simulink model "PQ_2V"  (R2023a)
settings: Solver=FixedStepAuto  StartTime=0.0  StopTime=10.0  FixedStep=Ts  RelTol=1e-3
InitFcn:
  | Ts = 1e-6;
  | Ikp = 0.1 ;
  | Iki = 0.002*12800 ;
  | 
  | Pref = 0;
  | Qref = 600e3;
libraries: slpidlib x4, spsabctodq0Lib x3, spsThreePhaseSeriesRLCBranchLib x2, spsThreePhaseVIMeasurementLib x1, spsDCVoltageSourceLib x1, powerlib_extras x1, spsGroundLib x1, spsMultimeterLib x1, spsPLL3phLib x1, spsPower3phInstantaneousLib x1, spsSeriesRLCBranchLib x1, spsThreePhaseSourceLib x1
settings Model: Creator=Cyril  LastModifiedBy=Cyril
settings SolverCC: AlgebraicLoopSolver=TrustRegion
settings DebuggingCC: UnconnectedInputMsg=warning  UnconnectedOutputMsg=warning  UnconnectedLineMsg=warning
settings ModelReferenceCC: EnableRefExpFcnMdlSchedulingChecks=on
settings RTWCC: DLArmComputeVersion=19.05

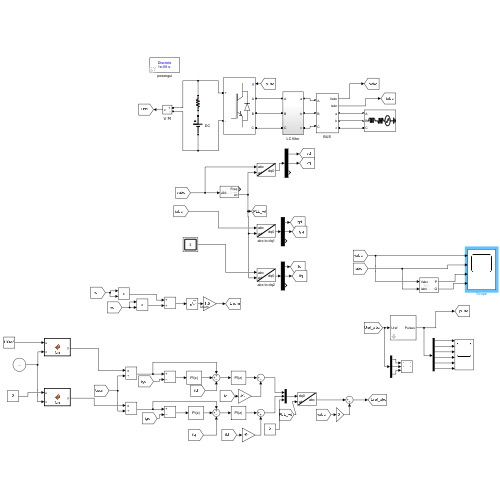
[thumbnail: Simulink's stored preview of the top-level diagram]
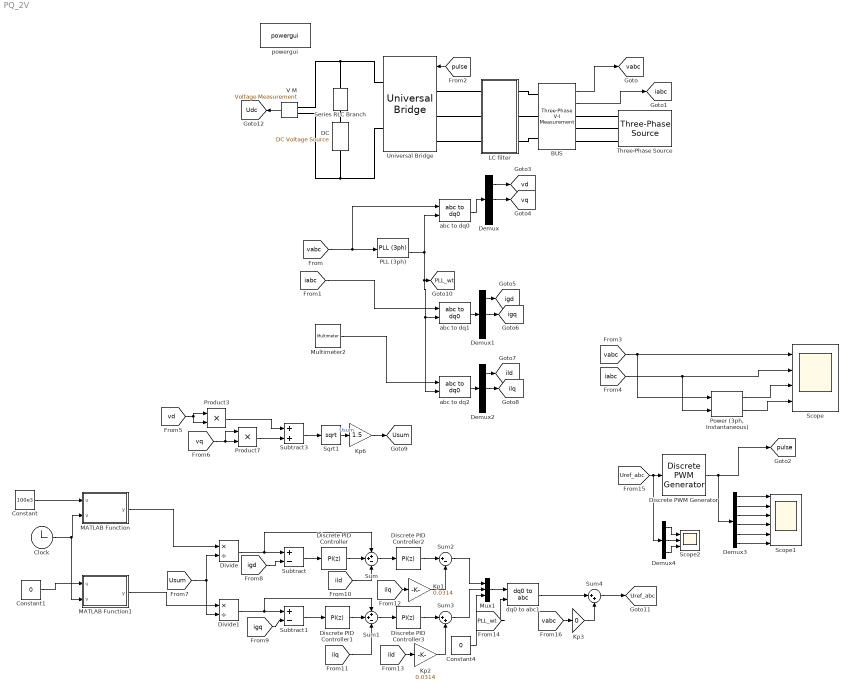
== system PQ_2V ==
  BUS : spsThreePhaseVIMeasurementLib/Three-Phase V-I Measurement  VoltageMeasurement=phase-to-ground  SetLabelV=off  LabelV=Vabc  Vpu=off  VpuLL=off  CurrentMeasurement=yes  SetLabelI=off  LabelI=Iabc  Ipu=off  Pbase=100e6  Vbase=500e3  OutputType=Complex  PhasorSimulation=off  PSBequivalent=0
  Clock : Clock
  Constant : Constant  Value=100e3  SampleTime=-1
  Constant1 : Constant  Value=0  SampleTime=-1
  Constant4 : Constant  Value=0
  "DC " : spsDCVoltageSourceLib/DC Voltage Source  Amplitude=800  Measurements=None
  Demux{,1..2,4} (4 alike) : Demux  Outputs=3
  Demux3 : Demux  Outputs=6
  Discrete PWM Generator : powerlib_extras/Discrete  Control Blocks/Discrete PWM Generator  GeneratorMode="3-arm  bridge (6 pulses)"  Fc=4266  Ts=Ts  Internal=off  mIndex=0.4  Freq=60  Phase=0
  Discrete PID Controller{,1..3} (4 alike) : slpidlib/PID Controller  Controller=PI  Form=Parallel  TimeDomain=Discrete-time  UseExternalTs=off  SampleTime=Ts  IntegratorMethod=Forward Euler  FilterMethod=Forward Euler  ControllerParametersSource=internal  P=Ikp  I=Iki  UseKiTs=off  D=0  N=100  UseFilter=on  TunerSelectOption=Transfer Function Based (PID Tuner App)  InitialConditionSource=internal  InitialConditionForIntegrator=0  InitialConditionForFilter=0  DifferentiatorICPrevScaledInput=0  ExternalReset=none  TrackingMode=off  Kt=1  LimitOutput=off  SatLimitsSource=internal  UpperSaturationLimit=inf  LowerSaturationLimit=-inf  LinearizeAsGain=off  AntiWindupMode=none  Kb=1  LimitIntegrator=off  UpperIntegratorSaturationLimit=inf  LowerIntegratorSaturationLimit=-inf  POutMin=[]  POutMax=[]  IOutMin=[]  IOutMax=[]  DOutMin=[]  DOutMax=[]  NOutMin=[]  NOutMax=[]  SumOutMin=[]  SumOutMax=[]  SaturationOutMin=[]  SaturationOutMax=[]  PParamMin=[]  PParamMax=[]  IParamMin=[]  IParamMax=[]  DParamMin=[]  DParamMax=[]  NParamMin=[]  NParamMax=[]  KbParamMin=[]  KbParamMax=[]  KtParamMin=[]  KtParamMax=[]  KbOutMin=[]  KbOutMax=[]  KtOutMin=[]  KtOutMax=[]  IntegratorOutMin=[]  IntegratorOutMax=[]  FilterOutMin=[]  FilterOutMax=[]  SumI1OutMin=[]  SumI1OutMax=[]  SumI2OutMin=[]  SumI2OutMax=[]  SumI3OutMin=[]  SumI3OutMax=[]  SumI4OutMin=[]  SumI4OutMax=[]  SumDOutMin=[]  SumDOutMax=[]  DifferentiatorOutMin=[]  DifferentiatorOutMax=[]  FilterDiffOutCoefMin=[]  FilterDiffOutCoefMax=[]  ReciprocalOutMin=[]  ReciprocalOutMax=[]  SumDenOutMin=[]  SumDenOutMax=[]  SumNumOutMin=[]  SumNumOutMax=[]  DivideOutMin=[]  DivideOutMax=[]  UdiffTsProdOutMin=[]  UdiffTsProdOutMax=[]  NTsProdOutMin=[]  NTsProdOutMax=[]  UintegralTsProdOutMin=[]  UintegralTsProdOutMax=[]  UngainTsProdOutMin=[]  UngainTsProdOutMax=[]  ClampingZeroOutDataTypeStr=Inherit: Inherit via back propagation  ClampingZeroOutMin=[]  ClampingZeroOutMax=[]  FilterDenConstantOutDataTypeStr=Inherit: Inherit via back propagation  FilterDenConstantOutMin=[]  FilterDenConstantOutMax=[]  PCopyOutDataTypeStr=Inherit: Inherit via back propagation  PCopyOutMin=[]  PCopyOutMax=[]  NCopyOutDataTypeStr=Inherit: Inherit via back propagation  NCopyOutMin=[]  NCopyOutMax=[]  IntegratorContinuousStateAttributes=''  IntegratorStateMustResolveToSignalObject=off  IntegratorRTWStateStorageClass=Auto  FilterContinuousStateAttributes=''  FilterStateMustResolveToSignalObject=off  FilterRTWStateStorageClass=Auto  ParallelPVariant=InternalParameters  IdealPVariant=Disabled  IVariant=InternalParameters  DVariant=Disabled  IntegratorVariant=Discrete  SatVariant=Disabled  AWVariant=Passthrough  PCopyVariant=Disabled  TRVariant=Disabled  FdbkBlocksVariant=Forward  IdealPFdbkVariant=Disabled  SatFdbkVariant=Disabled  DerivativeFilterVariant=Disabled  NVariant=Disabled  NCopyVariant=Disabled_SignalSpec  FilterICVariant=Disabled  IntegratorICVariant=InternalICs  ExternalResetVariant=Disabled  TRSumVariant=Passthrough  SumFdbkVariant=Disabled  SumVariant=Sum_PI  TsampFilterVariant=InternalTs  TsampNgainVariant=Passthrough  TsampIntegralVariant=Disabled_SignalSpec  ExternalSaturationOutDataTypeStr=Inherit: Same as second input
  Divide : Product  Inputs=*/
  Divide1 : Product  Inputs=*/
  Kp1 : Gain  Gain=0.0314  SaturateOnIntegerOverflow=on  OutDataTypeStr=Inherit: Same as input  ParamDataTypeStr=Inherit: Same as input
  Kp2 : Gain  Gain=0.0314  SaturateOnIntegerOverflow=on  OutDataTypeStr=Inherit: Same as input  ParamDataTypeStr=Inherit: Same as input
  Kp3 : Gain  Gain=0  SaturateOnIntegerOverflow=on  OutDataTypeStr=Inherit: Same as input  ParamDataTypeStr=Inherit: Same as input
  Kp6 : Gain  Gain=1.5  SaturateOnIntegerOverflow=on  OutDataTypeStr=Inherit: Same as input  ParamDataTypeStr=Inherit: Same as input
  LC filter : Subsystem
  MATLAB Function : MATLAB Function  TreatAsAtomicUnit=on
  MATLAB Function1 : MATLAB Function  TreatAsAtomicUnit=on
  Multimeter2 : spsMultimeterLib/Multimeter  L=3  sel=[1 2 3]  Gain=[1 1 1]  OutputType=Complex  PlotAtSimulationStop=off  PhasorSimulation=off
  Mux1 : Mux  Inputs=3
  PLL (3ph) : spsPLL3phLib/PLL (3ph)  Fmin=50  Par_Init=[0, 50]  ParK=[180, 3200, 1]  TcD=1e-5  MaxRateChangeFreq=12  FilterCutOffFreq=25  Ts=Ts  AGC=on
  "Power (3ph, Instantaneous)" : spsPower3phInstantaneousLib/Power (3ph, Instantaneous)
  Product3 : Product
  Product7 : Product
  Scope : Scope  NumInputPorts=4
  Scope1 : Scope  NumInputPorts=6
  Scope2 : Scope  NumInputPorts=3
  Series RLC Branch : spsSeriesRLCBranchLib/Series RLC Branch  LConnTagsString=__new0  RConnTagsString=__new0  BranchType=R  Resistance=1e-4  Inductance=1e-3  SetiL0=off  InitialCurrent=0  Capacitance=1e-6  Setx0=off  InitialVoltage=0  Measurements=None
  Sqrt1 : Sqrt
  Subtract : Sum  Inputs=+-
  Subtract1 : Sum  Inputs=+-
  Subtract3 : Sum
  Sum : Sum  Inputs=++-
  Sum1 : Sum  Inputs=++-
  Sum2 : Sum  Inputs=|+-
  Sum3 : Sum  Inputs=|++
  Sum4 : Sum  Inputs=|++
  Three-Phase Source : spsThreePhaseSourceLib/Three-Phase Source  InternalConnection=Yg  VoltagePhases=off  Voltage=380  PhaseAngle=0  Voltage_phases=[25e3 25e3 25e3]/sqrt(3)  PhaseAngles_phases=[0 -120 +120]  Frequency=50  NonIdealSource=on  SpecifyImpedance=on  Resistance=0.8929  Inductance=16.58e-3  ShortCircuitLevel=5000e6  BaseVoltage=380  XRratio=7  BusType=swing  Pref=0  Qref=0  Prefabc=[10e3, 10e3, 10e3]  Qrefabc=[0, 0, 0]  Qmin=-inf  Qmax=inf
  Universal Bridge : spsUniversalBridgeLib/Universal Bridge  Arms=3  SnubberResistance=1e5  SnubberCapacitance=inf  Device=IGBT / Diodes  Ron=1e-3  Lon=0  ForwardVoltages="[1  1]"  ForwardVoltage=0  GTOparameters=[ 10e-6 , 20e-6 ]  IGBTparameters=[ 1e-6 , 2e-6 ]  Measurements=None  Measurements_2=None  converterType=Rectifier
  V M : spsVoltageMeasurementLib/Voltage Measurement  PhasorSimulation=off  OutputType=Complex  PSBequivalent=0
  abc to dq0 : spsabctodq0Lib/abc to dq0  Alignment=90 degrees behind phase A axis
  abc to dq1 : spsabctodq0Lib/abc to dq0  Alignment=90 degrees behind phase A axis
  abc to dq2 : spsabctodq0Lib/abc to dq0  Alignment=90 degrees behind phase A axis
  dq0 to abc1 : spsdq0toabcLib/dq0 to abc  Alignment=90 degrees behind phase A axis
  powergui : sps_lib/powergui  Priority=1  SimulationMode=Discrete  SampleTime=Ts  frequency=60  Iterations=50  frequencyindice=50  Pbase=100e6  ErrMax=1e-4  UnitsV=kV  UnitsW=MW  buscounter=0  FunctionMessages=off  echomessages=off  EnableUseOfTLC=off  CurrentSourceSwitches=off  DisableSnubberDevices=off  DisableRonSwitches=off  DisableVfSwitches=off  DisplayEquations=off  AutomaticDiscreteSolvers=off  SolverType=Tustin/Backward Euler (TBE)  Interpol=off  ExternalGateDelay=off  methode=off  Ts=100  x0status=blocks  SPID=on  SwTol=0  HookPort=off  NonlinearTolerance=1e-4  nMaxIteration=100  ContinueOnMaxIteration=off  RestoreLinks=warning  ResistiveCurrentMeasurement=off  Frange=[0:2:500]  Ylog=off  Xlog=on  ShowGrid=off  save=off  variable=ZData  structure=0  ZoomFFT=off  StartTime=0.0  cycles=1  DisplayStyle=1  fundamental=60  FreqAxis=off  MaxFrequency=1000  frequencyindicesteady=1  RmsSteady=1  display=off
  tag scope: PLL_wt=global, Udc=global, Uref_abc=global, Usum=global, iabc=global, igd=global, igq=global, ild=global, ilq=global, pulse=global, vabc=global, vd=global, vq=global
  wires:
  BUS/1 -> [vabc]
  BUS/2 -> [iabc]
  [vabc] -> abc to dq0/1, PLL (3ph)/1
  PLL (3ph)/2 -> [PLL_wt], abc to dq2/2, abc to dq1/2, abc to dq0/2
  [iabc] -> abc to dq1/1
  Discrete PWM Generator/1 -> Demux3/1, [pulse]
  [pulse] -> Universal Bridge/1
  [vabc] -> "Power (3ph, Instantaneous)"/1, Scope/1
  [iabc] -> "Power (3ph, Instantaneous)"/2, Scope/2
  "Power (3ph, Instantaneous)"/1 -> Scope/3
  "Power (3ph, Instantaneous)"/2 -> Scope/4
  Multimeter2/1 -> abc to dq2/1
  abc to dq0/1 -> Demux/1
  Demux/1 -> [vd]
  Demux/2 -> [vq]
  abc to dq1/1 -> Demux1/1
  Demux1/1 -> [igd]
  Demux1/2 -> [igq]
  Demux2/2 -> [ilq]
  Demux2/1 -> [ild]
  abc to dq2/1 -> Demux2/1
  Subtract3/1 -> Sqrt1/1
  Product3/1 -> Subtract3/1
  Sqrt1/1 -> Kp6/1  "Usum"
  Product7/1 -> Subtract3/2
  [vd] -> Product3/2, Product3/1
  [vq] -> Product7/2, Product7/1
  Kp6/1 -> [Usum]
  [Usum] -> Divide/2, Divide1/2
  Divide/1 -> Sum/1, Subtract/1
  Divide1/1 -> Sum1/1, Subtract1/1
  [igd] -> Subtract/2
  [igq] -> Subtract1/2
  Subtract/1 -> Discrete PID Controller/1
  Subtract1/1 -> Discrete PID Controller1/1
  Discrete PID Controller/1 -> Sum/2
  [ild] -> Sum/3
  Discrete PID Controller1/1 -> Sum1/2
  [ilq] -> Sum1/3
  Sum/1 -> Discrete PID Controller2/1
  Sum1/1 -> Discrete PID Controller3/1
  Discrete PID Controller2/1 -> Sum2/1
  Discrete PID Controller3/1 -> Sum3/1
  [ilq] -> Kp1/1
  Kp1/1 -> Sum2/2
  [ild] -> Kp2/1
  Kp2/1 -> Sum3/2
  Sum2/1 -> Mux1/1
  Sum3/1 -> Mux1/2
  Constant4/1 -> Mux1/3
  Mux1/1 -> dq0 to abc1/1
  [PLL_wt] -> dq0 to abc1/2
  Clock/1 -> MATLAB Function1/2(v), MATLAB Function/2(v)
  Constant/1 -> MATLAB Function/1(u)
  Constant1/1 -> MATLAB Function1/1(u)
  MATLAB Function1/1(y) -> Divide1/1
  MATLAB Function/1(y) -> Divide/1
  Demux3/1 -> Scope1/1
  Demux3/2 -> Scope1/2
  Demux3/3 -> Scope1/3
  Demux3/4 -> Scope1/4
  Demux3/5 -> Scope1/5
  Demux3/6 -> Scope1/6
  V M/1 -> [Udc]
  Sum4/1 -> [Uref_abc]
  Demux4/2 -> Scope2/2
  Demux4/1 -> Scope2/1
  Demux4/3 -> Scope2/3
  [Uref_abc] -> Demux4/1, Discrete PWM Generator/1
  Kp3/1 -> Sum4/2
  dq0 to abc1/1 -> Sum4/1
  [vabc] -> Kp3/1
  connections:
  Universal Bridge/RConn2 -- "DC "/LConn1 -- V M/LConn2
  V M/LConn1 -- Series RLC Branch/LConn1 -- Universal Bridge/RConn1
  LC filter/LConn1 -- Universal Bridge/LConn1
  LC filter/LConn2 -- Universal Bridge/LConn2
  LC filter/LConn3 -- Universal Bridge/LConn3
  BUS/LConn2 -- LC filter/RConn2
  BUS/LConn1 -- LC filter/RConn1
  BUS/LConn3 -- LC filter/RConn3
  Three-Phase Source/RConn1 -- BUS/RConn1
  Three-Phase Source/RConn2 -- BUS/RConn2
  Three-Phase Source/RConn3 -- BUS/RConn3
  "DC "/RConn1 -- Series RLC Branch/RConn1

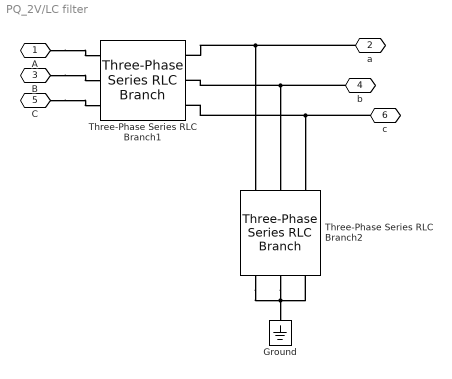
== system PQ_2V/LC filter ==
  Ground : spsGroundLib/Ground  LConnTagsString=a
  Three-Phase Series RLC Branch1 : spsThreePhaseSeriesRLCBranchLib/Three-Phase Series RLC Branch  LConnTagsString=A|B|C  RConnTagsString=A|B|C  BranchType=RL  Resistance=0.1e-6  Inductance=0.1e-3  Capacitance=inf  Measurements=Branch currents
  Three-Phase Series RLC Branch2 : spsThreePhaseSeriesRLCBranchLib/Three-Phase Series RLC Branch  LConnTagsString=A|B|C  RConnTagsString=A|B|C  BranchType=RC  Resistance=0.1e-6  Inductance=0  Capacitance=600e-6  Measurements=None
  A : PMIOPort  Side=Left
  a : PMIOPort  Port=2  Side=Right
  B : PMIOPort  Port=3  Side=Left
  b : PMIOPort  Port=4  Side=Right
  C : PMIOPort  Port=5  Side=Left
  c : PMIOPort  Port=6  Side=Right
  connections:
  A/RConn1 -- Three-Phase Series RLC Branch1/LConn1
  a/RConn1 -- Three-Phase Series RLC Branch1/RConn1 -- Three-Phase Series RLC Branch2/LConn1
  B/RConn1 -- Three-Phase Series RLC Branch1/LConn2
  b/RConn1 -- Three-Phase Series RLC Branch1/RConn2 -- Three-Phase Series RLC Branch2/LConn2
  C/RConn1 -- Three-Phase Series RLC Branch1/LConn3
  c/RConn1 -- Three-Phase Series RLC Branch1/RConn3 -- Three-Phase Series RLC Branch2/LConn3
  Three-Phase Series RLC Branch2/RConn1 -- Three-Phase Series RLC Branch2/RConn2 -- Three-Phase Series RLC Branch2/RConn3 -- Ground/LConn1

== matlab function PQ_2V/MATLAB Function ==
  data: u input; y output; v input
function y = fcn(u,v)
%#codegen
x = v*2 ;
if (x>1)
    x=1 ;
end

y = u*x;

== matlab function PQ_2V/MATLAB Function1 ==
  data: u input; y output; v input
function y = fcn(u,v)
%#codegen
x = v*2 ;
if (x>1)
    x=1 ;
end

y = u*x;
